simulink library "pack_105s34p_structured"  (R2023b)
settings: Solver=VariableStepAuto  StartTime=0.0  StopTime=10.0  RelTol=1e-3
undefined symbols (not defined in the file or in its folder): battery_builder_rtmsupport, gcbh
libraries: nesl_utility x156, pack_105s34p_structured_lib x156
(part 6 of 7)

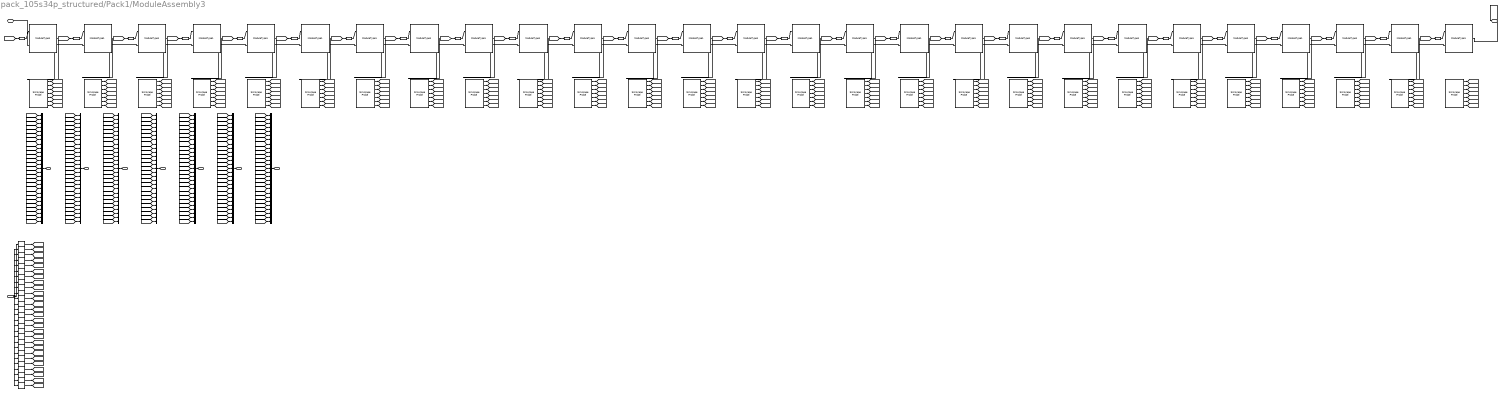
== system pack_105s34p_structured/Pack1/ModuleAssembly3 ==
  note: Balancing Signals
  note: Output Signals
  note: Battery Modules
  balancing : Inport  PortDimensions=27
  Converter{1..27} (27 alike) : nesl_utility/Simulink-PS Converter  PhysicalDomain=network_engine_domain  SubClassName=ps_input  LeftPortType=input  RightPortType=output  PseudoPeriodic=off  Frequencies=[]  NoiseDistribution=none  NoiseParameters=[]  Unit=1  AffineConversion=off  FilteringAndDerivatives=provide  SimscapeFilterOrder=1  InputFilterTimeConstant=0.001  UdotUserProvided=0
  Module01 : pack_105s34p_structured_lib/Modules/ModuleType1  SOC_vecCell=[0, .1, .25, .5, .75, .9, 1]  T_vecCell=[278, 293, 313] K  V0_matCell=[3.49, 3.5, 3.51; 3.55, 3.57, 3.56; 3.62, 3.63, 3.64; 3.71, 3.71, 3.72; 3.91, 3.93, 3.94; 4.07, 4.08, 4.08; 4.19, 4.19, 4.19] V  V_rangeCell=[0, inf] V  R0_matCell=[.0117, .0085, .009; .011, .0085, .009; .0114, .0087, .0092; .0107, .0082, .0088; .0107, .0083, .0091; .0113, .0085, .0089; .0116, .0085, .0089] Ohm  AHCell=4.9 A*hr  extrapolation_optionCell=simscape.enum.extrapolation.nearest  SOC_Init=0  R1_matCell=[.0109, .0029, .0013; .0069, .0024, .0012; .0047, .0026, .0013; .0034, .0016, .001; .0033, .0023, .0014; .0033, .0018, .0011; .0028, .0017, .0011] Ohm  tau1_matCell=[20, 36, 39; 31, 45, 39; 109, 105, 61; 36, 29, 26; 59, 77, 67; 40, 33, 29; 25, 39, 33] s  R2_matCell=[.0109, .0029, .0013; .0069, .0024, .0012; .0047, .0026, .0013; .0034, .0016, .001; .0033, .0023, .0014; .0033, .0018, .0011; .0028, .0017, .0011] Ohm  tau2_matCell=[20, 36, 39; 31, 45, 39; 109, 105, 61; 36, 29, 26; 59, 77, 67; 40, 33, 29; 25, 39, 33] s  R3_matCell=[.0109, .0029, .0013; .0069, .0024, .0012; .0047, .0026, .0013; .0034, .0016, .001; .0033, .0023, .0014; .0033, .0018, .0011; .0028, .0017, .0011] Ohm  tau3_matCell=[20, 36, 39; 31, 45, 39; 109, 105, 61; 36, 29, 26; 59, 77, 67; 40, 33, 29; 25, 39, 33] s  thermal_massCell=100 J/K  CellBalancingClosedResistance=0.01 Ohm  CellBalancingOpenConductance=1e-8 1/Ohm  CellBalancingThreshold=0.5  CellBalancingResistance=50 Ohm  P=34  S=1  iCell_specify=off  iCell_priority=None  iCell=0 A  iCell_nominal_specify=off  iCell_nominal_unit=A  iCell_nominal_value=1  vCell_specify=off  vCell_priority=None  vCell=0 V  vCell_nominal_specify=off  vCell_nominal_unit=V  vCell_nominal_value=1  numCyclesCell_specify=off  numCyclesCell_priority=High  numCyclesCell=0  numCyclesCell_nominal_specify=off  numCyclesCell_nominal_unit=1  numCyclesCell_nominal_value=1  temperatureCell_specify=off  temperatureCell_priority=High  temperatureCell=298.15 K  temperatureCell_nominal_specify=off  temperatureCell_nominal_unit=K  temperatureCell_nominal_value=1  vParallelAssembly_specify=off  vParallelAssembly_priority=None  vParallelAssembly=0 V  vParallelAssembly_nominal_specify=off  vParallelAssembly_nominal_unit=V  vParallelAssembly_nominal_value=1  socParallelAssembly_specify=off  socParallelAssembly_priority=None  socParallelAssembly=1  socParallelAssembly_nominal_specify=off  socParallelAssembly_nominal_unit=1  socParallelAssembly_nominal_value=1
      settings: InternalSimscapePortConfiguration="{\"Bottom\":[{\"id\":\"n\",\"label\":\"-\",\"type\":\"foundation.electrical.electrical\"}],\"Left\":[{\"id\":\"enableCellBalancing\",\"label\":\"CB\",\"type\":\"input\"}],\"Right\":[],\"Top\":[{\"id\":\"p\",\"label\":\"+\",\"type\":\"foundation.electrical.electrical\"}]}"
  Module01_outputs : SimscapeProbe  BoundBlock=2156  Variables={iCell, numCyclesCell, socCell, socParallelAssembly, temperatureCell, vCell, vParallelAssembly}
  Module02 : pack_105s34p_structured_lib/Modules/ModuleType1  SOC_vecCell=[0, .1, .25, .5, .75, .9, 1]  T_vecCell=[278, 293, 313] K  V0_matCell=[3.49, 3.5, 3.51; 3.55, 3.57, 3.56; 3.62, 3.63, 3.64; 3.71, 3.71, 3.72; 3.91, 3.93, 3.94; 4.07, 4.08, 4.08; 4.19, 4.19, 4.19] V  V_rangeCell=[0, inf] V  R0_matCell=[.0117, .0085, .009; .011, .0085, .009; .0114, .0087, .0092; .0107, .0082, .0088; .0107, .0083, .0091; .0113, .0085, .0089; .0116, .0085, .0089] Ohm  AHCell=4.9 A*hr  extrapolation_optionCell=simscape.enum.extrapolation.nearest  SOC_Init=0  R1_matCell=[.0109, .0029, .0013; .0069, .0024, .0012; .0047, .0026, .0013; .0034, .0016, .001; .0033, .0023, .0014; .0033, .0018, .0011; .0028, .0017, .0011] Ohm  tau1_matCell=[20, 36, 39; 31, 45, 39; 109, 105, 61; 36, 29, 26; 59, 77, 67; 40, 33, 29; 25, 39, 33] s  R2_matCell=[.0109, .0029, .0013; .0069, .0024, .0012; .0047, .0026, .0013; .0034, .0016, .001; .0033, .0023, .0014; .0033, .0018, .0011; .0028, .0017, .0011] Ohm  tau2_matCell=[20, 36, 39; 31, 45, 39; 109, 105, 61; 36, 29, 26; 59, 77, 67; 40, 33, 29; 25, 39, 33] s  R3_matCell=[.0109, .0029, .0013; .0069, .0024, .0012; .0047, .0026, .0013; .0034, .0016, .001; .0033, .0023, .0014; .0033, .0018, .0011; .0028, .0017, .0011] Ohm  tau3_matCell=[20, 36, 39; 31, 45, 39; 109, 105, 61; 36, 29, 26; 59, 77, 67; 40, 33, 29; 25, 39, 33] s  thermal_massCell=100 J/K  CellBalancingClosedResistance=0.01 Ohm  CellBalancingOpenConductance=1e-8 1/Ohm  CellBalancingThreshold=0.5  CellBalancingResistance=50 Ohm  P=34  S=1  iCell_specify=off  iCell_priority=None  iCell=0 A  iCell_nominal_specify=off  iCell_nominal_unit=A  iCell_nominal_value=1  vCell_specify=off  vCell_priority=None  vCell=0 V  vCell_nominal_specify=off  vCell_nominal_unit=V  vCell_nominal_value=1  numCyclesCell_specify=off  numCyclesCell_priority=High  numCyclesCell=0  numCyclesCell_nominal_specify=off  numCyclesCell_nominal_unit=1  numCyclesCell_nominal_value=1  temperatureCell_specify=off  temperatureCell_priority=High  temperatureCell=298.15 K  temperatureCell_nominal_specify=off  temperatureCell_nominal_unit=K  temperatureCell_nominal_value=1  vParallelAssembly_specify=off  vParallelAssembly_priority=None  vParallelAssembly=0 V  vParallelAssembly_nominal_specify=off  vParallelAssembly_nominal_unit=V  vParallelAssembly_nominal_value=1  socParallelAssembly_specify=off  socParallelAssembly_priority=None  socParallelAssembly=1  socParallelAssembly_nominal_specify=off  socParallelAssembly_nominal_unit=1  socParallelAssembly_nominal_value=1
      settings: InternalSimscapePortConfiguration="{\"Bottom\":[{\"id\":\"n\",\"label\":\"-\",\"type\":\"foundation.electrical.electrical\"}],\"Left\":[{\"id\":\"enableCellBalancing\",\"label\":\"CB\",\"type\":\"input\"}],\"Right\":[],\"Top\":[{\"id\":\"p\",\"label\":\"+\",\"type\":\"foundation.electrical.electrical\"}]}"
  Module02_outputs : SimscapeProbe  BoundBlock=2158  Variables={iCell, numCyclesCell, socCell, socParallelAssembly, temperatureCell, vCell, vParallelAssembly}
  Module03 : pack_105s34p_structured_lib/Modules/ModuleType1  SOC_vecCell=[0, .1, .25, .5, .75, .9, 1]  T_vecCell=[278, 293, 313] K  V0_matCell=[3.49, 3.5, 3.51; 3.55, 3.57, 3.56; 3.62, 3.63, 3.64; 3.71, 3.71, 3.72; 3.91, 3.93, 3.94; 4.07, 4.08, 4.08; 4.19, 4.19, 4.19] V  V_rangeCell=[0, inf] V  R0_matCell=[.0117, .0085, .009; .011, .0085, .009; .0114, .0087, .0092; .0107, .0082, .0088; .0107, .0083, .0091; .0113, .0085, .0089; .0116, .0085, .0089] Ohm  AHCell=4.9 A*hr  extrapolation_optionCell=simscape.enum.extrapolation.nearest  SOC_Init=0  R1_matCell=[.0109, .0029, .0013; .0069, .0024, .0012; .0047, .0026, .0013; .0034, .0016, .001; .0033, .0023, .0014; .0033, .0018, .0011; .0028, .0017, .0011] Ohm  tau1_matCell=[20, 36, 39; 31, 45, 39; 109, 105, 61; 36, 29, 26; 59, 77, 67; 40, 33, 29; 25, 39, 33] s  R2_matCell=[.0109, .0029, .0013; .0069, .0024, .0012; .0047, .0026, .0013; .0034, .0016, .001; .0033, .0023, .0014; .0033, .0018, .0011; .0028, .0017, .0011] Ohm  tau2_matCell=[20, 36, 39; 31, 45, 39; 109, 105, 61; 36, 29, 26; 59, 77, 67; 40, 33, 29; 25, 39, 33] s  R3_matCell=[.0109, .0029, .0013; .0069, .0024, .0012; .0047, .0026, .0013; .0034, .0016, .001; .0033, .0023, .0014; .0033, .0018, .0011; .0028, .0017, .0011] Ohm  tau3_matCell=[20, 36, 39; 31, 45, 39; 109, 105, 61; 36, 29, 26; 59, 77, 67; 40, 33, 29; 25, 39, 33] s  thermal_massCell=100 J/K  CellBalancingClosedResistance=0.01 Ohm  CellBalancingOpenConductance=1e-8 1/Ohm  CellBalancingThreshold=0.5  CellBalancingResistance=50 Ohm  P=34  S=1  iCell_specify=off  iCell_priority=None  iCell=0 A  iCell_nominal_specify=off  iCell_nominal_unit=A  iCell_nominal_value=1  vCell_specify=off  vCell_priority=None  vCell=0 V  vCell_nominal_specify=off  vCell_nominal_unit=V  vCell_nominal_value=1  numCyclesCell_specify=off  numCyclesCell_priority=High  numCyclesCell=0  numCyclesCell_nominal_specify=off  numCyclesCell_nominal_unit=1  numCyclesCell_nominal_value=1  temperatureCell_specify=off  temperatureCell_priority=High  temperatureCell=298.15 K  temperatureCell_nominal_specify=off  temperatureCell_nominal_unit=K  temperatureCell_nominal_value=1  vParallelAssembly_specify=off  vParallelAssembly_priority=None  vParallelAssembly=0 V  vParallelAssembly_nominal_specify=off  vParallelAssembly_nominal_unit=V  vParallelAssembly_nominal_value=1  socParallelAssembly_specify=off  socParallelAssembly_priority=None  socParallelAssembly=1  socParallelAssembly_nominal_specify=off  socParallelAssembly_nominal_unit=1  socParallelAssembly_nominal_value=1
      settings: InternalSimscapePortConfiguration="{\"Bottom\":[{\"id\":\"n\",\"label\":\"-\",\"type\":\"foundation.electrical.electrical\"}],\"Left\":[{\"id\":\"enableCellBalancing\",\"label\":\"CB\",\"type\":\"input\"}],\"Right\":[],\"Top\":[{\"id\":\"p\",\"label\":\"+\",\"type\":\"foundation.electrical.electrical\"}]}"
  Module03_outputs : SimscapeProbe  BoundBlock=2160  Variables={iCell, numCyclesCell, socCell, socParallelAssembly, temperatureCell, vCell, vParallelAssembly}
  Module04 : pack_105s34p_structured_lib/Modules/ModuleType1  SOC_vecCell=[0, .1, .25, .5, .75, .9, 1]  T_vecCell=[278, 293, 313] K  V0_matCell=[3.49, 3.5, 3.51; 3.55, 3.57, 3.56; 3.62, 3.63, 3.64; 3.71, 3.71, 3.72; 3.91, 3.93, 3.94; 4.07, 4.08, 4.08; 4.19, 4.19, 4.19] V  V_rangeCell=[0, inf] V  R0_matCell=[.0117, .0085, .009; .011, .0085, .009; .0114, .0087, .0092; .0107, .0082, .0088; .0107, .0083, .0091; .0113, .0085, .0089; .0116, .0085, .0089] Ohm  AHCell=4.9 A*hr  extrapolation_optionCell=simscape.enum.extrapolation.nearest  SOC_Init=0  R1_matCell=[.0109, .0029, .0013; .0069, .0024, .0012; .0047, .0026, .0013; .0034, .0016, .001; .0033, .0023, .0014; .0033, .0018, .0011; .0028, .0017, .0011] Ohm  tau1_matCell=[20, 36, 39; 31, 45, 39; 109, 105, 61; 36, 29, 26; 59, 77, 67; 40, 33, 29; 25, 39, 33] s  R2_matCell=[.0109, .0029, .0013; .0069, .0024, .0012; .0047, .0026, .0013; .0034, .0016, .001; .0033, .0023, .0014; .0033, .0018, .0011; .0028, .0017, .0011] Ohm  tau2_matCell=[20, 36, 39; 31, 45, 39; 109, 105, 61; 36, 29, 26; 59, 77, 67; 40, 33, 29; 25, 39, 33] s  R3_matCell=[.0109, .0029, .0013; .0069, .0024, .0012; .0047, .0026, .0013; .0034, .0016, .001; .0033, .0023, .0014; .0033, .0018, .0011; .0028, .0017, .0011] Ohm  tau3_matCell=[20, 36, 39; 31, 45, 39; 109, 105, 61; 36, 29, 26; 59, 77, 67; 40, 33, 29; 25, 39, 33] s  thermal_massCell=100 J/K  CellBalancingClosedResistance=0.01 Ohm  CellBalancingOpenConductance=1e-8 1/Ohm  CellBalancingThreshold=0.5  CellBalancingResistance=50 Ohm  P=34  S=1  iCell_specify=off  iCell_priority=None  iCell=0 A  iCell_nominal_specify=off  iCell_nominal_unit=A  iCell_nominal_value=1  vCell_specify=off  vCell_priority=None  vCell=0 V  vCell_nominal_specify=off  vCell_nominal_unit=V  vCell_nominal_value=1  numCyclesCell_specify=off  numCyclesCell_priority=High  numCyclesCell=0  numCyclesCell_nominal_specify=off  numCyclesCell_nominal_unit=1  numCyclesCell_nominal_value=1  temperatureCell_specify=off  temperatureCell_priority=High  temperatureCell=298.15 K  temperatureCell_nominal_specify=off  temperatureCell_nominal_unit=K  temperatureCell_nominal_value=1  vParallelAssembly_specify=off  vParallelAssembly_priority=None  vParallelAssembly=0 V  vParallelAssembly_nominal_specify=off  vParallelAssembly_nominal_unit=V  vParallelAssembly_nominal_value=1  socParallelAssembly_specify=off  socParallelAssembly_priority=None  socParallelAssembly=1  socParallelAssembly_nominal_specify=off  socParallelAssembly_nominal_unit=1  socParallelAssembly_nominal_value=1
      settings: InternalSimscapePortConfiguration="{\"Bottom\":[{\"id\":\"n\",\"label\":\"-\",\"type\":\"foundation.electrical.electrical\"}],\"Left\":[{\"id\":\"enableCellBalancing\",\"label\":\"CB\",\"type\":\"input\"}],\"Right\":[],\"Top\":[{\"id\":\"p\",\"label\":\"+\",\"type\":\"foundation.electrical.electrical\"}]}"
  Module04_outputs : SimscapeProbe  BoundBlock=2162  Variables={iCell, numCyclesCell, socCell, socParallelAssembly, temperatureCell, vCell, vParallelAssembly}
  Module05 : pack_105s34p_structured_lib/Modules/ModuleType1  SOC_vecCell=[0, .1, .25, .5, .75, .9, 1]  T_vecCell=[278, 293, 313] K  V0_matCell=[3.49, 3.5, 3.51; 3.55, 3.57, 3.56; 3.62, 3.63, 3.64; 3.71, 3.71, 3.72; 3.91, 3.93, 3.94; 4.07, 4.08, 4.08; 4.19, 4.19, 4.19] V  V_rangeCell=[0, inf] V  R0_matCell=[.0117, .0085, .009; .011, .0085, .009; .0114, .0087, .0092; .0107, .0082, .0088; .0107, .0083, .0091; .0113, .0085, .0089; .0116, .0085, .0089] Ohm  AHCell=4.9 A*hr  extrapolation_optionCell=simscape.enum.extrapolation.nearest  SOC_Init=0  R1_matCell=[.0109, .0029, .0013; .0069, .0024, .0012; .0047, .0026, .0013; .0034, .0016, .001; .0033, .0023, .0014; .0033, .0018, .0011; .0028, .0017, .0011] Ohm  tau1_matCell=[20, 36, 39; 31, 45, 39; 109, 105, 61; 36, 29, 26; 59, 77, 67; 40, 33, 29; 25, 39, 33] s  R2_matCell=[.0109, .0029, .0013; .0069, .0024, .0012; .0047, .0026, .0013; .0034, .0016, .001; .0033, .0023, .0014; .0033, .0018, .0011; .0028, .0017, .0011] Ohm  tau2_matCell=[20, 36, 39; 31, 45, 39; 109, 105, 61; 36, 29, 26; 59, 77, 67; 40, 33, 29; 25, 39, 33] s  R3_matCell=[.0109, .0029, .0013; .0069, .0024, .0012; .0047, .0026, .0013; .0034, .0016, .001; .0033, .0023, .0014; .0033, .0018, .0011; .0028, .0017, .0011] Ohm  tau3_matCell=[20, 36, 39; 31, 45, 39; 109, 105, 61; 36, 29, 26; 59, 77, 67; 40, 33, 29; 25, 39, 33] s  thermal_massCell=100 J/K  CellBalancingClosedResistance=0.01 Ohm  CellBalancingOpenConductance=1e-8 1/Ohm  CellBalancingThreshold=0.5  CellBalancingResistance=50 Ohm  P=34  S=1  iCell_specify=off  iCell_priority=None  iCell=0 A  iCell_nominal_specify=off  iCell_nominal_unit=A  iCell_nominal_value=1  vCell_specify=off  vCell_priority=None  vCell=0 V  vCell_nominal_specify=off  vCell_nominal_unit=V  vCell_nominal_value=1  numCyclesCell_specify=off  numCyclesCell_priority=High  numCyclesCell=0  numCyclesCell_nominal_specify=off  numCyclesCell_nominal_unit=1  numCyclesCell_nominal_value=1  temperatureCell_specify=off  temperatureCell_priority=High  temperatureCell=298.15 K  temperatureCell_nominal_specify=off  temperatureCell_nominal_unit=K  temperatureCell_nominal_value=1  vParallelAssembly_specify=off  vParallelAssembly_priority=None  vParallelAssembly=0 V  vParallelAssembly_nominal_specify=off  vParallelAssembly_nominal_unit=V  vParallelAssembly_nominal_value=1  socParallelAssembly_specify=off  socParallelAssembly_priority=None  socParallelAssembly=1  socParallelAssembly_nominal_specify=off  socParallelAssembly_nominal_unit=1  socParallelAssembly_nominal_value=1
      settings: InternalSimscapePortConfiguration="{\"Bottom\":[{\"id\":\"n\",\"label\":\"-\",\"type\":\"foundation.electrical.electrical\"}],\"Left\":[{\"id\":\"enableCellBalancing\",\"label\":\"CB\",\"type\":\"input\"}],\"Right\":[],\"Top\":[{\"id\":\"p\",\"label\":\"+\",\"type\":\"foundation.electrical.electrical\"}]}"
  Module05_outputs : SimscapeProbe  BoundBlock=2164  Variables={iCell, numCyclesCell, socCell, socParallelAssembly, temperatureCell, vCell, vParallelAssembly}
  Module06 : pack_105s34p_structured_lib/Modules/ModuleType1  SOC_vecCell=[0, .1, .25, .5, .75, .9, 1]  T_vecCell=[278, 293, 313] K  V0_matCell=[3.49, 3.5, 3.51; 3.55, 3.57, 3.56; 3.62, 3.63, 3.64; 3.71, 3.71, 3.72; 3.91, 3.93, 3.94; 4.07, 4.08, 4.08; 4.19, 4.19, 4.19] V  V_rangeCell=[0, inf] V  R0_matCell=[.0117, .0085, .009; .011, .0085, .009; .0114, .0087, .0092; .0107, .0082, .0088; .0107, .0083, .0091; .0113, .0085, .0089; .0116, .0085, .0089] Ohm  AHCell=4.9 A*hr  extrapolation_optionCell=simscape.enum.extrapolation.nearest  SOC_Init=0  R1_matCell=[.0109, .0029, .0013; .0069, .0024, .0012; .0047, .0026, .0013; .0034, .0016, .001; .0033, .0023, .0014; .0033, .0018, .0011; .0028, .0017, .0011] Ohm  tau1_matCell=[20, 36, 39; 31, 45, 39; 109, 105, 61; 36, 29, 26; 59, 77, 67; 40, 33, 29; 25, 39, 33] s  R2_matCell=[.0109, .0029, .0013; .0069, .0024, .0012; .0047, .0026, .0013; .0034, .0016, .001; .0033, .0023, .0014; .0033, .0018, .0011; .0028, .0017, .0011] Ohm  tau2_matCell=[20, 36, 39; 31, 45, 39; 109, 105, 61; 36, 29, 26; 59, 77, 67; 40, 33, 29; 25, 39, 33] s  R3_matCell=[.0109, .0029, .0013; .0069, .0024, .0012; .0047, .0026, .0013; .0034, .0016, .001; .0033, .0023, .0014; .0033, .0018, .0011; .0028, .0017, .0011] Ohm  tau3_matCell=[20, 36, 39; 31, 45, 39; 109, 105, 61; 36, 29, 26; 59, 77, 67; 40, 33, 29; 25, 39, 33] s  thermal_massCell=100 J/K  CellBalancingClosedResistance=0.01 Ohm  CellBalancingOpenConductance=1e-8 1/Ohm  CellBalancingThreshold=0.5  CellBalancingResistance=50 Ohm  P=34  S=1  iCell_specify=off  iCell_priority=None  iCell=0 A  iCell_nominal_specify=off  iCell_nominal_unit=A  iCell_nominal_value=1  vCell_specify=off  vCell_priority=None  vCell=0 V  vCell_nominal_specify=off  vCell_nominal_unit=V  vCell_nominal_value=1  numCyclesCell_specify=off  numCyclesCell_priority=High  numCyclesCell=0  numCyclesCell_nominal_specify=off  numCyclesCell_nominal_unit=1  numCyclesCell_nominal_value=1  temperatureCell_specify=off  temperatureCell_priority=High  temperatureCell=298.15 K  temperatureCell_nominal_specify=off  temperatureCell_nominal_unit=K  temperatureCell_nominal_value=1  vParallelAssembly_specify=off  vParallelAssembly_priority=None  vParallelAssembly=0 V  vParallelAssembly_nominal_specify=off  vParallelAssembly_nominal_unit=V  vParallelAssembly_nominal_value=1  socParallelAssembly_specify=off  socParallelAssembly_priority=None  socParallelAssembly=1  socParallelAssembly_nominal_specify=off  socParallelAssembly_nominal_unit=1  socParallelAssembly_nominal_value=1
      settings: InternalSimscapePortConfiguration="{\"Bottom\":[{\"id\":\"n\",\"label\":\"-\",\"type\":\"foundation.electrical.electrical\"}],\"Left\":[{\"id\":\"enableCellBalancing\",\"label\":\"CB\",\"type\":\"input\"}],\"Right\":[],\"Top\":[{\"id\":\"p\",\"label\":\"+\",\"type\":\"foundation.electrical.electrical\"}]}"
  Module06_outputs : SimscapeProbe  BoundBlock=2166  Variables={iCell, numCyclesCell, socCell, socParallelAssembly, temperatureCell, vCell, vParallelAssembly}
  Module07 : pack_105s34p_structured_lib/Modules/ModuleType1  SOC_vecCell=[0, .1, .25, .5, .75, .9, 1]  T_vecCell=[278, 293, 313] K  V0_matCell=[3.49, 3.5, 3.51; 3.55, 3.57, 3.56; 3.62, 3.63, 3.64; 3.71, 3.71, 3.72; 3.91, 3.93, 3.94; 4.07, 4.08, 4.08; 4.19, 4.19, 4.19] V  V_rangeCell=[0, inf] V  R0_matCell=[.0117, .0085, .009; .011, .0085, .009; .0114, .0087, .0092; .0107, .0082, .0088; .0107, .0083, .0091; .0113, .0085, .0089; .0116, .0085, .0089] Ohm  AHCell=4.9 A*hr  extrapolation_optionCell=simscape.enum.extrapolation.nearest  SOC_Init=0  R1_matCell=[.0109, .0029, .0013; .0069, .0024, .0012; .0047, .0026, .0013; .0034, .0016, .001; .0033, .0023, .0014; .0033, .0018, .0011; .0028, .0017, .0011] Ohm  tau1_matCell=[20, 36, 39; 31, 45, 39; 109, 105, 61; 36, 29, 26; 59, 77, 67; 40, 33, 29; 25, 39, 33] s  R2_matCell=[.0109, .0029, .0013; .0069, .0024, .0012; .0047, .0026, .0013; .0034, .0016, .001; .0033, .0023, .0014; .0033, .0018, .0011; .0028, .0017, .0011] Ohm  tau2_matCell=[20, 36, 39; 31, 45, 39; 109, 105, 61; 36, 29, 26; 59, 77, 67; 40, 33, 29; 25, 39, 33] s  R3_matCell=[.0109, .0029, .0013; .0069, .0024, .0012; .0047, .0026, .0013; .0034, .0016, .001; .0033, .0023, .0014; .0033, .0018, .0011; .0028, .0017, .0011] Ohm  tau3_matCell=[20, 36, 39; 31, 45, 39; 109, 105, 61; 36, 29, 26; 59, 77, 67; 40, 33, 29; 25, 39, 33] s  thermal_massCell=100 J/K  CellBalancingClosedResistance=0.01 Ohm  CellBalancingOpenConductance=1e-8 1/Ohm  CellBalancingThreshold=0.5  CellBalancingResistance=50 Ohm  P=34  S=1  iCell_specify=off  iCell_priority=None  iCell=0 A  iCell_nominal_specify=off  iCell_nominal_unit=A  iCell_nominal_value=1  vCell_specify=off  vCell_priority=None  vCell=0 V  vCell_nominal_specify=off  vCell_nominal_unit=V  vCell_nominal_value=1  numCyclesCell_specify=off  numCyclesCell_priority=High  numCyclesCell=0  numCyclesCell_nominal_specify=off  numCyclesCell_nominal_unit=1  numCyclesCell_nominal_value=1  temperatureCell_specify=off  temperatureCell_priority=High  temperatureCell=298.15 K  temperatureCell_nominal_specify=off  temperatureCell_nominal_unit=K  temperatureCell_nominal_value=1  vParallelAssembly_specify=off  vParallelAssembly_priority=None  vParallelAssembly=0 V  vParallelAssembly_nominal_specify=off  vParallelAssembly_nominal_unit=V  vParallelAssembly_nominal_value=1  socParallelAssembly_specify=off  socParallelAssembly_priority=None  socParallelAssembly=1  socParallelAssembly_nominal_specify=off  socParallelAssembly_nominal_unit=1  socParallelAssembly_nominal_value=1
      settings: InternalSimscapePortConfiguration="{\"Bottom\":[{\"id\":\"n\",\"label\":\"-\",\"type\":\"foundation.electrical.electrical\"}],\"Left\":[{\"id\":\"enableCellBalancing\",\"label\":\"CB\",\"type\":\"input\"}],\"Right\":[],\"Top\":[{\"id\":\"p\",\"label\":\"+\",\"type\":\"foundation.electrical.electrical\"}]}"
  Module07_outputs : SimscapeProbe  BoundBlock=2168  Variables={iCell, numCyclesCell, socCell, socParallelAssembly, temperatureCell, vCell, vParallelAssembly}
  Module08 : pack_105s34p_structured_lib/Modules/ModuleType1  SOC_vecCell=[0, .1, .25, .5, .75, .9, 1]  T_vecCell=[278, 293, 313] K  V0_matCell=[3.49, 3.5, 3.51; 3.55, 3.57, 3.56; 3.62, 3.63, 3.64; 3.71, 3.71, 3.72; 3.91, 3.93, 3.94; 4.07, 4.08, 4.08; 4.19, 4.19, 4.19] V  V_rangeCell=[0, inf] V  R0_matCell=[.0117, .0085, .009; .011, .0085, .009; .0114, .0087, .0092; .0107, .0082, .0088; .0107, .0083, .0091; .0113, .0085, .0089; .0116, .0085, .0089] Ohm  AHCell=4.9 A*hr  extrapolation_optionCell=simscape.enum.extrapolation.nearest  SOC_Init=0  R1_matCell=[.0109, .0029, .0013; .0069, .0024, .0012; .0047, .0026, .0013; .0034, .0016, .001; .0033, .0023, .0014; .0033, .0018, .0011; .0028, .0017, .0011] Ohm  tau1_matCell=[20, 36, 39; 31, 45, 39; 109, 105, 61; 36, 29, 26; 59, 77, 67; 40, 33, 29; 25, 39, 33] s  R2_matCell=[.0109, .0029, .0013; .0069, .0024, .0012; .0047, .0026, .0013; .0034, .0016, .001; .0033, .0023, .0014; .0033, .0018, .0011; .0028, .0017, .0011] Ohm  tau2_matCell=[20, 36, 39; 31, 45, 39; 109, 105, 61; 36, 29, 26; 59, 77, 67; 40, 33, 29; 25, 39, 33] s  R3_matCell=[.0109, .0029, .0013; .0069, .0024, .0012; .0047, .0026, .0013; .0034, .0016, .001; .0033, .0023, .0014; .0033, .0018, .0011; .0028, .0017, .0011] Ohm  tau3_matCell=[20, 36, 39; 31, 45, 39; 109, 105, 61; 36, 29, 26; 59, 77, 67; 40, 33, 29; 25, 39, 33] s  thermal_massCell=100 J/K  CellBalancingClosedResistance=0.01 Ohm  CellBalancingOpenConductance=1e-8 1/Ohm  CellBalancingThreshold=0.5  CellBalancingResistance=50 Ohm  P=34  S=1  iCell_specify=off  iCell_priority=None  iCell=0 A  iCell_nominal_specify=off  iCell_nominal_unit=A  iCell_nominal_value=1  vCell_specify=off  vCell_priority=None  vCell=0 V  vCell_nominal_specify=off  vCell_nominal_unit=V  vCell_nominal_value=1  numCyclesCell_specify=off  numCyclesCell_priority=High  numCyclesCell=0  numCyclesCell_nominal_specify=off  numCyclesCell_nominal_unit=1  numCyclesCell_nominal_value=1  temperatureCell_specify=off  temperatureCell_priority=High  temperatureCell=298.15 K  temperatureCell_nominal_specify=off  temperatureCell_nominal_unit=K  temperatureCell_nominal_value=1  vParallelAssembly_specify=off  vParallelAssembly_priority=None  vParallelAssembly=0 V  vParallelAssembly_nominal_specify=off  vParallelAssembly_nominal_unit=V  vParallelAssembly_nominal_value=1  socParallelAssembly_specify=off  socParallelAssembly_priority=None  socParallelAssembly=1  socParallelAssembly_nominal_specify=off  socParallelAssembly_nominal_unit=1  socParallelAssembly_nominal_value=1
      settings: InternalSimscapePortConfiguration="{\"Bottom\":[{\"id\":\"n\",\"label\":\"-\",\"type\":\"foundation.electrical.electrical\"}],\"Left\":[{\"id\":\"enableCellBalancing\",\"label\":\"CB\",\"type\":\"input\"}],\"Right\":[],\"Top\":[{\"id\":\"p\",\"label\":\"+\",\"type\":\"foundation.electrical.electrical\"}]}"
  Module08_outputs : SimscapeProbe  BoundBlock=2170  Variables={iCell, numCyclesCell, socCell, socParallelAssembly, temperatureCell, vCell, vParallelAssembly}
  Module09 : pack_105s34p_structured_lib/Modules/ModuleType1  SOC_vecCell=[0, .1, .25, .5, .75, .9, 1]  T_vecCell=[278, 293, 313] K  V0_matCell=[3.49, 3.5, 3.51; 3.55, 3.57, 3.56; 3.62, 3.63, 3.64; 3.71, 3.71, 3.72; 3.91, 3.93, 3.94; 4.07, 4.08, 4.08; 4.19, 4.19, 4.19] V  V_rangeCell=[0, inf] V  R0_matCell=[.0117, .0085, .009; .011, .0085, .009; .0114, .0087, .0092; .0107, .0082, .0088; .0107, .0083, .0091; .0113, .0085, .0089; .0116, .0085, .0089] Ohm  AHCell=4.9 A*hr  extrapolation_optionCell=simscape.enum.extrapolation.nearest  SOC_Init=0  R1_matCell=[.0109, .0029, .0013; .0069, .0024, .0012; .0047, .0026, .0013; .0034, .0016, .001; .0033, .0023, .0014; .0033, .0018, .0011; .0028, .0017, .0011] Ohm  tau1_matCell=[20, 36, 39; 31, 45, 39; 109, 105, 61; 36, 29, 26; 59, 77, 67; 40, 33, 29; 25, 39, 33] s  R2_matCell=[.0109, .0029, .0013; .0069, .0024, .0012; .0047, .0026, .0013; .0034, .0016, .001; .0033, .0023, .0014; .0033, .0018, .0011; .0028, .0017, .0011] Ohm  tau2_matCell=[20, 36, 39; 31, 45, 39; 109, 105, 61; 36, 29, 26; 59, 77, 67; 40, 33, 29; 25, 39, 33] s  R3_matCell=[.0109, .0029, .0013; .0069, .0024, .0012; .0047, .0026, .0013; .0034, .0016, .001; .0033, .0023, .0014; .0033, .0018, .0011; .0028, .0017, .0011] Ohm  tau3_matCell=[20, 36, 39; 31, 45, 39; 109, 105, 61; 36, 29, 26; 59, 77, 67; 40, 33, 29; 25, 39, 33] s  thermal_massCell=100 J/K  CellBalancingClosedResistance=0.01 Ohm  CellBalancingOpenConductance=1e-8 1/Ohm  CellBalancingThreshold=0.5  CellBalancingResistance=50 Ohm  P=34  S=1  iCell_specify=off  iCell_priority=None  iCell=0 A  iCell_nominal_specify=off  iCell_nominal_unit=A  iCell_nominal_value=1  vCell_specify=off  vCell_priority=None  vCell=0 V  vCell_nominal_specify=off  vCell_nominal_unit=V  vCell_nominal_value=1  numCyclesCell_specify=off  numCyclesCell_priority=High  numCyclesCell=0  numCyclesCell_nominal_specify=off  numCyclesCell_nominal_unit=1  numCyclesCell_nominal_value=1  temperatureCell_specify=off  temperatureCell_priority=High  temperatureCell=298.15 K  temperatureCell_nominal_specify=off  temperatureCell_nominal_unit=K  temperatureCell_nominal_value=1  vParallelAssembly_specify=off  vParallelAssembly_priority=None  vParallelAssembly=0 V  vParallelAssembly_nominal_specify=off  vParallelAssembly_nominal_unit=V  vParallelAssembly_nominal_value=1  socParallelAssembly_specify=off  socParallelAssembly_priority=None  socParallelAssembly=1  socParallelAssembly_nominal_specify=off  socParallelAssembly_nominal_unit=1  socParallelAssembly_nominal_value=1
      settings: InternalSimscapePortConfiguration="{\"Bottom\":[{\"id\":\"n\",\"label\":\"-\",\"type\":\"foundation.electrical.electrical\"}],\"Left\":[{\"id\":\"enableCellBalancing\",\"label\":\"CB\",\"type\":\"input\"}],\"Right\":[],\"Top\":[{\"id\":\"p\",\"label\":\"+\",\"type\":\"foundation.electrical.electrical\"}]}"
  Module09_outputs : SimscapeProbe  BoundBlock=2172  Variables={iCell, numCyclesCell, socCell, socParallelAssembly, temperatureCell, vCell, vParallelAssembly}
  Module{10..27} (18 alike) : pack_105s34p_structured_lib/Modules/ModuleType1  SOC_vecCell=[0, .1, .25, .5, .75, .9, 1]  T_vecCell=[278, 293, 313] K  V0_matCell=[3.49, 3.5, 3.51; 3.55, 3.57, 3.56; 3.62, 3.63, 3.64; 3.71, 3.71, 3.72; 3.91, 3.93, 3.94; 4.07, 4.08, 4.08; 4.19, 4.19, 4.19] V  V_rangeCell=[0, inf] V  R0_matCell=[.0117, .0085, .009; .011, .0085, .009; .0114, .0087, .0092; .0107, .0082, .0088; .0107, .0083, .0091; .0113, .0085, .0089; .0116, .0085, .0089] Ohm  AHCell=4.9 A*hr  extrapolation_optionCell=simscape.enum.extrapolation.nearest  SOC_Init=0  R1_matCell=[.0109, .0029, .0013; .0069, .0024, .0012; .0047, .0026, .0013; .0034, .0016, .001; .0033, .0023, .0014; .0033, .0018, .0011; .0028, .0017, .0011] Ohm  tau1_matCell=[20, 36, 39; 31, 45, 39; 109, 105, 61; 36, 29, 26; 59, 77, 67; 40, 33, 29; 25, 39, 33] s  R2_matCell=[.0109, .0029, .0013; .0069, .0024, .0012; .0047, .0026, .0013; .0034, .0016, .001; .0033, .0023, .0014; .0033, .0018, .0011; .0028, .0017, .0011] Ohm  tau2_matCell=[20, 36, 39; 31, 45, 39; 109, 105, 61; 36, 29, 26; 59, 77, 67; 40, 33, 29; 25, 39, 33] s  R3_matCell=[.0109, .0029, .0013; .0069, .0024, .0012; .0047, .0026, .0013; .0034, .0016, .001; .0033, .0023, .0014; .0033, .0018, .0011; .0028, .0017, .0011] Ohm  tau3_matCell=[20, 36, 39; 31, 45, 39; 109, 105, 61; 36, 29, 26; 59, 77, 67; 40, 33, 29; 25, 39, 33] s  thermal_massCell=100 J/K  CellBalancingClosedResistance=0.01 Ohm  CellBalancingOpenConductance=1e-8 1/Ohm  CellBalancingThreshold=0.5  CellBalancingResistance=50 Ohm  P=34  S=1  iCell_specify=off  iCell_priority=None  iCell=0 A  iCell_nominal_specify=off  iCell_nominal_unit=A  iCell_nominal_value=1  vCell_specify=off  vCell_priority=None  vCell=0 V  vCell_nominal_specify=off  vCell_nominal_unit=V  vCell_nominal_value=1  numCyclesCell_specify=off  numCyclesCell_priority=High  numCyclesCell=0  numCyclesCell_nominal_specify=off  numCyclesCell_nominal_unit=1  numCyclesCell_nominal_value=1  temperatureCell_specify=off  temperatureCell_priority=High  temperatureCell=298.15 K  temperatureCell_nominal_specify=off  temperatureCell_nominal_unit=K  temperatureCell_nominal_value=1  vParallelAssembly_specify=off  vParallelAssembly_priority=None  vParallelAssembly=0 V  vParallelAssembly_nominal_specify=off  vParallelAssembly_nominal_unit=V  vParallelAssembly_nominal_value=1  socParallelAssembly_specify=off  socParallelAssembly_priority=None  socParallelAssembly=1  socParallelAssembly_nominal_specify=off  socParallelAssembly_nominal_unit=1  socParallelAssembly_nominal_value=1
      settings: InternalSimscapePortConfiguration="{\"Bottom\":[{\"id\":\"n\",\"label\":\"-\",\"type\":\"foundation.electrical.electrical\"}],\"Left\":[{\"id\":\"enableCellBalancing\",\"label\":\"CB\",\"type\":\"input\"}],\"Right\":[],\"Top\":[{\"id\":\"p\",\"label\":\"+\",\"type\":\"foundation.electrical.electrical\"}]}"
  Module10_outputs : SimscapeProbe  BoundBlock=2174  Variables={iCell, numCyclesCell, socCell, socParallelAssembly, temperatureCell, vCell, vParallelAssembly}
  Module11_outputs : SimscapeProbe  BoundBlock=2176  Variables={iCell, numCyclesCell, socCell, socParallelAssembly, temperatureCell, vCell, vParallelAssembly}
  Module12_outputs : SimscapeProbe  BoundBlock=2178  Variables={iCell, numCyclesCell, socCell, socParallelAssembly, temperatureCell, vCell, vParallelAssembly}
  Module13_outputs : SimscapeProbe  BoundBlock=2180  Variables={iCell, numCyclesCell, socCell, socParallelAssembly, temperatureCell, vCell, vParallelAssembly}
  Module14_outputs : SimscapeProbe  BoundBlock=2182  Variables={iCell, numCyclesCell, socCell, socParallelAssembly, temperatureCell, vCell, vParallelAssembly}
  Module15_outputs : SimscapeProbe  BoundBlock=2184  Variables={iCell, numCyclesCell, socCell, socParallelAssembly, temperatureCell, vCell, vParallelAssembly}
  Module16_outputs : SimscapeProbe  BoundBlock=2186  Variables={iCell, numCyclesCell, socCell, socParallelAssembly, temperatureCell, vCell, vParallelAssembly}
  Module17_outputs : SimscapeProbe  BoundBlock=2188  Variables={iCell, numCyclesCell, socCell, socParallelAssembly, temperatureCell, vCell, vParallelAssembly}
  Module18_outputs : SimscapeProbe  BoundBlock=2190  Variables={iCell, numCyclesCell, socCell, socParallelAssembly, temperatureCell, vCell, vParallelAssembly}
  Module19_outputs : SimscapeProbe  BoundBlock=2192  Variables={iCell, numCyclesCell, socCell, socParallelAssembly, temperatureCell, vCell, vParallelAssembly}
  Module20_outputs : SimscapeProbe  BoundBlock=2194  Variables={iCell, numCyclesCell, socCell, socParallelAssembly, temperatureCell, vCell, vParallelAssembly}
  Module21_outputs : SimscapeProbe  BoundBlock=2196  Variables={iCell, numCyclesCell, socCell, socParallelAssembly, temperatureCell, vCell, vParallelAssembly}
  Module22_outputs : SimscapeProbe  BoundBlock=2198  Variables={iCell, numCyclesCell, socCell, socParallelAssembly, temperatureCell, vCell, vParallelAssembly}
  Module23_outputs : SimscapeProbe  BoundBlock=2200  Variables={iCell, numCyclesCell, socCell, socParallelAssembly, temperatureCell, vCell, vParallelAssembly}
  Module24_outputs : SimscapeProbe  BoundBlock=2202  Variables={iCell, numCyclesCell, socCell, socParallelAssembly, temperatureCell, vCell, vParallelAssembly}
  Module25_outputs : SimscapeProbe  BoundBlock=2204  Variables={iCell, numCyclesCell, socCell, socParallelAssembly, temperatureCell, vCell, vParallelAssembly}
  Module26_outputs : SimscapeProbe  BoundBlock=2206  Variables={iCell, numCyclesCell, socCell, socParallelAssembly, temperatureCell, vCell, vParallelAssembly}
  Module27_outputs : SimscapeProbe  BoundBlock=2208  Variables={iCell, numCyclesCell, socCell, socParallelAssembly, temperatureCell, vCell, vParallelAssembly}
  balancingSelector1 : Selector  InputPortWidth=27  IndexOptions=Index vector (dialog)  Indices=[1]  OutputSizes=1
  balancingSelector10 : Selector  InputPortWidth=27  IndexOptions=Index vector (dialog)  Indices=[10]  OutputSizes=1
  balancingSelector11 : Selector  InputPortWidth=27  IndexOptions=Index vector (dialog)  Indices=[11]  OutputSizes=1
  balancingSelector12 : Selector  InputPortWidth=27  IndexOptions=Index vector (dialog)  Indices=[12]  OutputSizes=1
  balancingSelector13 : Selector  InputPortWidth=27  IndexOptions=Index vector (dialog)  Indices=[13]  OutputSizes=1
  balancingSelector14 : Selector  InputPortWidth=27  IndexOptions=Index vector (dialog)  Indices=[14]  OutputSizes=1
  balancingSelector15 : Selector  InputPortWidth=27  IndexOptions=Index vector (dialog)  Indices=[15]  OutputSizes=1
  balancingSelector16 : Selector  InputPortWidth=27  IndexOptions=Index vector (dialog)  Indices=[16]  OutputSizes=1
  balancingSelector17 : Selector  InputPortWidth=27  IndexOptions=Index vector (dialog)  Indices=[17]  OutputSizes=1
  balancingSelector18 : Selector  InputPortWidth=27  IndexOptions=Index vector (dialog)  Indices=[18]  OutputSizes=1
  balancingSelector19 : Selector  InputPortWidth=27  IndexOptions=Index vector (dialog)  Indices=[19]  OutputSizes=1
  balancingSelector2 : Selector  InputPortWidth=27  IndexOptions=Index vector (dialog)  Indices=[2]  OutputSizes=1
  balancingSelector20 : Selector  InputPortWidth=27  IndexOptions=Index vector (dialog)  Indices=[20]  OutputSizes=1
  balancingSelector21 : Selector  InputPortWidth=27  IndexOptions=Index vector (dialog)  Indices=[21]  OutputSizes=1
  balancingSelector22 : Selector  InputPortWidth=27  IndexOptions=Index vector (dialog)  Indices=[22]  OutputSizes=1
  balancingSelector23 : Selector  InputPortWidth=27  IndexOptions=Index vector (dialog)  Indices=[23]  OutputSizes=1
  balancingSelector24 : Selector  InputPortWidth=27  IndexOptions=Index vector (dialog)  Indices=[24]  OutputSizes=1
  balancingSelector25 : Selector  InputPortWidth=27  IndexOptions=Index vector (dialog)  Indices=[25]  OutputSizes=1
  balancingSelector26 : Selector  InputPortWidth=27  IndexOptions=Index vector (dialog)  Indices=[26]  OutputSizes=1
  balancingSelector27 : Selector  InputPortWidth=27  IndexOptions=Index vector (dialog)  Indices=[27]  OutputSizes=1
  balancingSelector3 : Selector  InputPortWidth=27  IndexOptions=Index vector (dialog)  Indices=[3]  OutputSizes=1
  balancingSelector4 : Selector  InputPortWidth=27  IndexOptions=Index vector (dialog)  Indices=[4]  OutputSizes=1
  balancingSelector5 : Selector  InputPortWidth=27  IndexOptions=Index vector (dialog)  Indices=[5]  OutputSizes=1
  balancingSelector6 : Selector  InputPortWidth=27  IndexOptions=Index vector (dialog)  Indices=[6]  OutputSizes=1
  balancingSelector7 : Selector  InputPortWidth=27  IndexOptions=Index vector (dialog)  Indices=[7]  OutputSizes=1
  balancingSelector8 : Selector  InputPortWidth=27  IndexOptions=Index vector (dialog)  Indices=[8]  OutputSizes=1
  balancingSelector9 : Selector  InputPortWidth=27  IndexOptions=Index vector (dialog)  Indices=[9]  OutputSizes=1
  iCellMux : Mux  Inputs=27
  numCyclesCellMux : Mux  Inputs=27
  socCellMux : Mux  Inputs=27
  socParallelAssemblyMux : Mux  Inputs=27
  temperatureCellMux : Mux  Inputs=27
  vCellMux : Mux  Inputs=27
  vParallelAssemblyMux : Mux  Inputs=27
  + : PMIOPort  Side=Left
  - : PMIOPort  Port=2  Side=Right
  iCell : Outport
  numCyclesCell : Outport  Port=2
  socCell : Outport  Port=3
  socParallelAssembly : Outport  Port=4
  temperatureCell : Outport  Port=5
  vCell : Outport  Port=6
  vParallelAssembly : Outport  Port=7
  wires:
  balancingSelector27/1 -> [balancing27]
  [balancing27] -> Converter27/1
  balancingSelector26/1 -> [balancing26]
  [balancing26] -> Converter26/1
  balancingSelector25/1 -> [balancing25]
  [balancing25] -> Converter25/1
  balancingSelector24/1 -> [balancing24]
  [balancing24] -> Converter24/1
  balancingSelector23/1 -> [balancing23]
  [balancing23] -> Converter23/1
  balancingSelector22/1 -> [balancing22]
  [balancing22] -> Converter22/1
  balancingSelector21/1 -> [balancing21]
  [balancing21] -> Converter21/1
  balancingSelector20/1 -> [balancing20]
  [balancing20] -> Converter20/1
  balancingSelector19/1 -> [balancing19]
  [balancing19] -> Converter19/1
  balancingSelector18/1 -> [balancing18]
  [balancing18] -> Converter18/1
  balancingSelector17/1 -> [balancing17]
  [balancing17] -> Converter17/1
  balancingSelector16/1 -> [balancing16]
  [balancing16] -> Converter16/1
  balancingSelector15/1 -> [balancing15]
  [balancing15] -> Converter15/1
  balancingSelector14/1 -> [balancing14]
  [balancing14] -> Converter14/1
  balancingSelector13/1 -> [balancing13]
  [balancing13] -> Converter13/1
  balancingSelector12/1 -> [balancing12]
  [balancing12] -> Converter12/1
  balancingSelector11/1 -> [balancing11]
  [balancing11] -> Converter11/1
  balancingSelector10/1 -> [balancing10]
  [balancing10] -> Converter10/1
  balancingSelector9/1 -> [balancing9]
  [balancing9] -> Converter9/1
  balancingSelector8/1 -> [balancing8]
  [balancing8] -> Converter8/1
  balancingSelector7/1 -> [balancing7]
  [balancing7] -> Converter7/1
  balancingSelector6/1 -> [balancing6]
  [balancing6] -> Converter6/1
  balancingSelector5/1 -> [balancing5]
  [balancing5] -> Converter5/1
  balancingSelector4/1 -> [balancing4]
  [balancing4] -> Converter4/1
  balancingSelector3/1 -> [balancing3]
  [balancing3] -> Converter3/1
  balancingSelector2/1 -> [balancing2]
  [balancing2] -> Converter2/1
  balancingSelector1/1 -> [balancing1]
  balancing/1 -> balancingSelector27/1, balancingSelector26/1, balancingSelector25/1, balancingSelector24/1, balancingSelector23/1, balancingSelector22/1, balancingSelector21/1, balancingSelector20/1, balancingSelector19/1, balancingSelector18/1, balancingSelector17/1, balancingSelector16/1, balancingSelector15/1, balancingSelector14/1, balancingSelector13/1, balancingSelector12/1, balancingSelector11/1, balancingSelector10/1, balancingSelector9/1, balancingSelector8/1, balancingSelector7/1, balancingSelector6/1, balancingSelector5/1, balancingSelector4/1, balancingSelector3/1, balancingSelector2/1, balancingSelector1/1
  [balancing1] -> Converter1/1
  [vParallelAssembly27] -> vParallelAssemblyMux/27
  Module27_outputs/7 -> [vParallelAssembly27]
  [vCell27] -> vCellMux/27
  Module27_outputs/6 -> [vCell27]
  [temperatureCell27] -> temperatureCellMux/27
  Module27_outputs/5 -> [temperatureCell27]
  [socParallelAssembly27] -> socParallelAssemblyMux/27
  Module27_outputs/4 -> [socParallelAssembly27]
  [socCell27] -> socCellMux/27
  Module27_outputs/3 -> [socCell27]
  [numCyclesCell27] -> numCyclesCellMux/27
  Module27_outputs/2 -> [numCyclesCell27]
  [iCell27] -> iCellMux/27
  Module27_outputs/1 -> [iCell27]
  [vParallelAssembly26] -> vParallelAssemblyMux/26
  Module26_outputs/7 -> [vParallelAssembly26]
  [vCell26] -> vCellMux/26
  Module26_outputs/6 -> [vCell26]
  [temperatureCell26] -> temperatureCellMux/26
  Module26_outputs/5 -> [temperatureCell26]
  [socParallelAssembly26] -> socParallelAssemblyMux/26
  Module26_outputs/4 -> [socParallelAssembly26]
  [socCell26] -> socCellMux/26
  Module26_outputs/3 -> [socCell26]
  [numCyclesCell26] -> numCyclesCellMux/26
  Module26_outputs/2 -> [numCyclesCell26]
  [iCell26] -> iCellMux/26
  Module26_outputs/1 -> [iCell26]
  [vParallelAssembly25] -> vParallelAssemblyMux/25
  Module25_outputs/7 -> [vParallelAssembly25]
  [vCell25] -> vCellMux/25
  Module25_outputs/6 -> [vCell25]
  [temperatureCell25] -> temperatureCellMux/25
  Module25_outputs/5 -> [temperatureCell25]
  [socParallelAssembly25] -> socParallelAssemblyMux/25
  Module25_outputs/4 -> [socParallelAssembly25]
  [socCell25] -> socCellMux/25
  Module25_outputs/3 -> [socCell25]
  [numCyclesCell25] -> numCyclesCellMux/25
  Module25_outputs/2 -> [numCyclesCell25]
  [iCell25] -> iCellMux/25
  Module25_outputs/1 -> [iCell25]
  [vParallelAssembly24] -> vParallelAssemblyMux/24
  Module24_outputs/7 -> [vParallelAssembly24]
  [vCell24] -> vCellMux/24
  Module24_outputs/6 -> [vCell24]
  [temperatureCell24] -> temperatureCellMux/24
  Module24_outputs/5 -> [temperatureCell24]
  [socParallelAssembly24] -> socParallelAssemblyMux/24
  Module24_outputs/4 -> [socParallelAssembly24]
  [socCell24] -> socCellMux/24
  Module24_outputs/3 -> [socCell24]
  [numCyclesCell24] -> numCyclesCellMux/24
  Module24_outputs/2 -> [numCyclesCell24]
  [iCell24] -> iCellMux/24
  Module24_outputs/1 -> [iCell24]
  [vParallelAssembly23] -> vParallelAssemblyMux/23
  Module23_outputs/7 -> [vParallelAssembly23]
  [vCell23] -> vCellMux/23
  Module23_outputs/6 -> [vCell23]
  [temperatureCell23] -> temperatureCellMux/23
  Module23_outputs/5 -> [temperatureCell23]
  [socParallelAssembly23] -> socParallelAssemblyMux/23
  Module23_outputs/4 -> [socParallelAssembly23]
  [socCell23] -> socCellMux/23
  Module23_outputs/3 -> [socCell23]
  [numCyclesCell23] -> numCyclesCellMux/23
  Module23_outputs/2 -> [numCyclesCell23]
  [iCell23] -> iCellMux/23
  Module23_outputs/1 -> [iCell23]
  [vParallelAssembly22] -> vParallelAssemblyMux/22
  Module22_outputs/7 -> [vParallelAssembly22]
  [vCell22] -> vCellMux/22
  Module22_outputs/6 -> [vCell22]
  [temperatureCell22] -> temperatureCellMux/22
  Module22_outputs/5 -> [temperatureCell22]
  [socParallelAssembly22] -> socParallelAssemblyMux/22
  Module22_outputs/4 -> [socParallelAssembly22]
  [socCell22] -> socCellMux/22
  Module22_outputs/3 -> [socCell22]
  [numCyclesCell22] -> numCyclesCellMux/22
  Module22_outputs/2 -> [numCyclesCell22]
  [iCell22] -> iCellMux/22
  Module22_outputs/1 -> [iCell22]
  [vParallelAssembly21] -> vParallelAssemblyMux/21
  Module21_outputs/7 -> [vParallelAssembly21]
  [vCell21] -> vCellMux/21
  Module21_outputs/6 -> [vCell21]
  [temperatureCell21] -> temperatureCellMux/21
  Module21_outputs/5 -> [temperatureCell21]
  [socParallelAssembly21] -> socParallelAssemblyMux/21
  Module21_outputs/4 -> [socParallelAssembly21]
  [socCell21] -> socCellMux/21
  Module21_outputs/3 -> [socCell21]
  [numCyclesCell21] -> numCyclesCellMux/21
  Module21_outputs/2 -> [numCyclesCell21]
  [iCell21] -> iCellMux/21
  Module21_outputs/1 -> [iCell21]
  [vParallelAssembly20] -> vParallelAssemblyMux/20
  Module20_outputs/7 -> [vParallelAssembly20]
  [vCell20] -> vCellMux/20
  Module20_outputs/6 -> [vCell20]
  [temperatureCell20] -> temperatureCellMux/20
  Module20_outputs/5 -> [temperatureCell20]
  [socParallelAssembly20] -> socParallelAssemblyMux/20
  Module20_outputs/4 -> [socParallelAssembly20]
  [socCell20] -> socCellMux/20
  Module20_outputs/3 -> [socCell20]
  [numCyclesCell20] -> numCyclesCellMux/20
  Module20_outputs/2 -> [numCyclesCell20]
  [iCell20] -> iCellMux/20
  Module20_outputs/1 -> [iCell20]
  [vParallelAssembly19] -> vParallelAssemblyMux/19
  Module19_outputs/7 -> [vParallelAssembly19]
  [vCell19] -> vCellMux/19
  Module19_outputs/6 -> [vCell19]
  [temperatureCell19] -> temperatureCellMux/19
  Module19_outputs/5 -> [temperatureCell19]
  [socParallelAssembly19] -> socParallelAssemblyMux/19
  Module19_outputs/4 -> [socParallelAssembly19]
  [socCell19] -> socCellMux/19
  Module19_outputs/3 -> [socCell19]
  [numCyclesCell19] -> numCyclesCellMux/19
  Module19_outputs/2 -> [numCyclesCell19]
  [iCell19] -> iCellMux/19
  Module19_outputs/1 -> [iCell19]
  [vParallelAssembly18] -> vParallelAssemblyMux/18
  Module18_outputs/7 -> [vParallelAssembly18]
  [vCell18] -> vCellMux/18
  Module18_outputs/6 -> [vCell18]
  [temperatureCell18] -> temperatureCellMux/18
  Module18_outputs/5 -> [temperatureCell18]
  [socParallelAssembly18] -> socParallelAssemblyMux/18
  Module18_outputs/4 -> [socParallelAssembly18]
  [socCell18] -> socCellMux/18
  Module18_outputs/3 -> [socCell18]
  [numCyclesCell18] -> numCyclesCellMux/18
  Module18_outputs/2 -> [numCyclesCell18]
  [iCell18] -> iCellMux/18
  Module18_outputs/1 -> [iCell18]
  [vParallelAssembly17] -> vParallelAssemblyMux/17
  Module17_outputs/7 -> [vParallelAssembly17]
  [vCell17] -> vCellMux/17
  Module17_outputs/6 -> [vCell17]
  [temperatureCell17] -> temperatureCellMux/17
  Module17_outputs/5 -> [temperatureCell17]
  [socParallelAssembly17] -> socParallelAssemblyMux/17
  Module17_outputs/4 -> [socParallelAssembly17]
  [socCell17] -> socCellMux/17
  Module17_outputs/3 -> [socCell17]
  [numCyclesCell17] -> numCyclesCellMux/17
  Module17_outputs/2 -> [numCyclesCell17]
  [iCell17] -> iCellMux/17
  Module17_outputs/1 -> [iCell17]
  [vParallelAssembly16] -> vParallelAssemblyMux/16
  Module16_outputs/7 -> [vParallelAssembly16]
  [vCell16] -> vCellMux/16
  Module16_outputs/6 -> [vCell16]
  [temperatureCell16] -> temperatureCellMux/16
  Module16_outputs/5 -> [temperatureCell16]
  [socParallelAssembly16] -> socParallelAssemblyMux/16
  Module16_outputs/4 -> [socParallelAssembly16]
  [socCell16] -> socCellMux/16
  Module16_outputs/3 -> [socCell16]
  [numCyclesCell16] -> numCyclesCellMux/16
  Module16_outputs/2 -> [numCyclesCell16]
  [iCell16] -> iCellMux/16
  Module16_outputs/1 -> [iCell16]
  [vParallelAssembly15] -> vParallelAssemblyMux/15
  Module15_outputs/7 -> [vParallelAssembly15]
  [vCell15] -> vCellMux/15
  Module15_outputs/6 -> [vCell15]
  [temperatureCell15] -> temperatureCellMux/15
  Module15_outputs/5 -> [temperatureCell15]
  [socParallelAssembly15] -> socParallelAssemblyMux/15
  Module15_outputs/4 -> [socParallelAssembly15]
  [socCell15] -> socCellMux/15
  Module15_outputs/3 -> [socCell15]
  [numCyclesCell15] -> numCyclesCellMux/15
  Module15_outputs/2 -> [numCyclesCell15]
  [iCell15] -> iCellMux/15
  Module15_outputs/1 -> [iCell15]
  [vParallelAssembly14] -> vParallelAssemblyMux/14
  Module14_outputs/7 -> [vParallelAssembly14]
  [vCell14] -> vCellMux/14
  Module14_outputs/6 -> [vCell14]
  [temperatureCell14] -> temperatureCellMux/14
  Module14_outputs/5 -> [temperatureCell14]
  [socParallelAssembly14] -> socParallelAssemblyMux/14
  Module14_outputs/4 -> [socParallelAssembly14]
  [socCell14] -> socCellMux/14
  Module14_outputs/3 -> [socCell14]
  [numCyclesCell14] -> numCyclesCellMux/14
  Module14_outputs/2 -> [numCyclesCell14]
  [iCell14] -> iCellMux/14
  Module14_outputs/1 -> [iCell14]
  [vParallelAssembly13] -> vParallelAssemblyMux/13
  Module13_outputs/7 -> [vParallelAssembly13]
  [vCell13] -> vCellMux/13
  Module13_outputs/6 -> [vCell13]
  [temperatureCell13] -> temperatureCellMux/13
  Module13_outputs/5 -> [temperatureCell13]
  [socParallelAssembly13] -> socParallelAssemblyMux/13
  Module13_outputs/4 -> [socParallelAssembly13]
  [socCell13] -> socCellMux/13
  Module13_outputs/3 -> [socCell13]
  [numCyclesCell13] -> numCyclesCellMux/13
  Module13_outputs/2 -> [numCyclesCell13]
  [iCell13] -> iCellMux/13
  Module13_outputs/1 -> [iCell13]
  [vParallelAssembly12] -> vParallelAssemblyMux/12
  Module12_outputs/7 -> [vParallelAssembly12]
  [vCell12] -> vCellMux/12
  Module12_outputs/6 -> [vCell12]
  [temperatureCell12] -> temperatureCellMux/12
  Module12_outputs/5 -> [temperatureCell12]
  [socParallelAssembly12] -> socParallelAssemblyMux/12
  Module12_outputs/4 -> [socParallelAssembly12]
  [socCell12] -> socCellMux/12
  Module12_outputs/3 -> [socCell12]
  [numCyclesCell12] -> numCyclesCellMux/12
  Module12_outputs/2 -> [numCyclesCell12]
  [iCell12] -> iCellMux/12
  Module12_outputs/1 -> [iCell12]
  [vParallelAssembly11] -> vParallelAssemblyMux/11
  Module11_outputs/7 -> [vParallelAssembly11]
  [vCell11] -> vCellMux/11
  Module11_outputs/6 -> [vCell11]
  [temperatureCell11] -> temperatureCellMux/11
  Module11_outputs/5 -> [temperatureCell11]
  [socParallelAssembly11] -> socParallelAssemblyMux/11
  Module11_outputs/4 -> [socParallelAssembly11]
  [socCell11] -> socCellMux/11
  Module11_outputs/3 -> [socCell11]
  [numCyclesCell11] -> numCyclesCellMux/11
  Module11_outputs/2 -> [numCyclesCell11]
  [iCell11] -> iCellMux/11
  Module11_outputs/1 -> [iCell11]
  [vParallelAssembly10] -> vParallelAssemblyMux/10
  Module10_outputs/7 -> [vParallelAssembly10]
  [vCell10] -> vCellMux/10
  Module10_outputs/6 -> [vCell10]
  [temperatureCell10] -> temperatureCellMux/10
  Module10_outputs/5 -> [temperatureCell10]
  [socParallelAssembly10] -> socParallelAssemblyMux/10
  Module10_outputs/4 -> [socParallelAssembly10]
  [socCell10] -> socCellMux/10
  Module10_outputs/3 -> [socCell10]
  [numCyclesCell10] -> numCyclesCellMux/10
  Module10_outputs/2 -> [numCyclesCell10]
  [iCell10] -> iCellMux/10
  Module10_outputs/1 -> [iCell10]
  [vParallelAssembly9] -> vParallelAssemblyMux/9
  Module09_outputs/7 -> [vParallelAssembly9]
  [vCell9] -> vCellMux/9
  Module09_outputs/6 -> [vCell9]
  [temperatureCell9] -> temperatureCellMux/9
  Module09_outputs/5 -> [temperatureCell9]
  [socParallelAssembly9] -> socParallelAssemblyMux/9
  Module09_outputs/4 -> [socParallelAssembly9]
  [socCell9] -> socCellMux/9
  Module09_outputs/3 -> [socCell9]
  [numCyclesCell9] -> numCyclesCellMux/9
  Module09_outputs/2 -> [numCyclesCell9]
  [iCell9] -> iCellMux/9
  Module09_outputs/1 -> [iCell9]
  [vParallelAssembly8] -> vParallelAssemblyMux/8
  Module08_outputs/7 -> [vParallelAssembly8]
  [vCell8] -> vCellMux/8
  Module08_outputs/6 -> [vCell8]
  [temperatureCell8] -> temperatureCellMux/8
  Module08_outputs/5 -> [temperatureCell8]
  [socParallelAssembly8] -> socParallelAssemblyMux/8
  Module08_outputs/4 -> [socParallelAssembly8]
  [socCell8] -> socCellMux/8
  Module08_outputs/3 -> [socCell8]
  [numCyclesCell8] -> numCyclesCellMux/8
  Module08_outputs/2 -> [numCyclesCell8]
  [iCell8] -> iCellMux/8
  Module08_outputs/1 -> [iCell8]
  [vParallelAssembly7] -> vParallelAssemblyMux/7
  Module07_outputs/7 -> [vParallelAssembly7]
  [vCell7] -> vCellMux/7
  Module07_outputs/6 -> [vCell7]
  [temperatureCell7] -> temperatureCellMux/7
  Module07_outputs/5 -> [temperatureCell7]
  [socParallelAssembly7] -> socParallelAssemblyMux/7
  Module07_outputs/4 -> [socParallelAssembly7]
  [socCell7] -> socCellMux/7
  Module07_outputs/3 -> [socCell7]
  [numCyclesCell7] -> numCyclesCellMux/7
  Module07_outputs/2 -> [numCyclesCell7]
  [iCell7] -> iCellMux/7
  Module07_outputs/1 -> [iCell7]
  [vParallelAssembly6] -> vParallelAssemblyMux/6
  Module06_outputs/7 -> [vParallelAssembly6]
  [vCell6] -> vCellMux/6
  Module06_outputs/6 -> [vCell6]
  [temperatureCell6] -> temperatureCellMux/6
  Module06_outputs/5 -> [temperatureCell6]
  [socParallelAssembly6] -> socParallelAssemblyMux/6
  Module06_outputs/4 -> [socParallelAssembly6]
  [socCell6] -> socCellMux/6
  Module06_outputs/3 -> [socCell6]
  [numCyclesCell6] -> numCyclesCellMux/6
  Module06_outputs/2 -> [numCyclesCell6]
  [iCell6] -> iCellMux/6
  Module06_outputs/1 -> [iCell6]
  [vParallelAssembly5] -> vParallelAssemblyMux/5
  Module05_outputs/7 -> [vParallelAssembly5]
  [vCell5] -> vCellMux/5
  Module05_outputs/6 -> [vCell5]
  [temperatureCell5] -> temperatureCellMux/5
  Module05_outputs/5 -> [temperatureCell5]
  [socParallelAssembly5] -> socParallelAssemblyMux/5
  Module05_outputs/4 -> [socParallelAssembly5]
  [socCell5] -> socCellMux/5
  Module05_outputs/3 -> [socCell5]
  [numCyclesCell5] -> numCyclesCellMux/5
  Module05_outputs/2 -> [numCyclesCell5]
  [iCell5] -> iCellMux/5
  Module05_outputs/1 -> [iCell5]
  [vParallelAssembly4] -> vParallelAssemblyMux/4
  Module04_outputs/7 -> [vParallelAssembly4]
  [vCell4] -> vCellMux/4
  Module04_outputs/6 -> [vCell4]
  [temperatureCell4] -> temperatureCellMux/4
  Module04_outputs/5 -> [temperatureCell4]
  [socParallelAssembly4] -> socParallelAssemblyMux/4
  Module04_outputs/4 -> [socParallelAssembly4]
  [socCell4] -> socCellMux/4
  Module04_outputs/3 -> [socCell4]
  [numCyclesCell4] -> numCyclesCellMux/4
  Module04_outputs/2 -> [numCyclesCell4]
  [iCell4] -> iCellMux/4
  Module04_outputs/1 -> [iCell4]
  [vParallelAssembly3] -> vParallelAssemblyMux/3
  Module03_outputs/7 -> [vParallelAssembly3]
  [vCell3] -> vCellMux/3
  Module03_outputs/6 -> [vCell3]
  [temperatureCell3] -> temperatureCellMux/3
  Module03_outputs/5 -> [temperatureCell3]
  [socParallelAssembly3] -> socParallelAssemblyMux/3
  Module03_outputs/4 -> [socParallelAssembly3]
  [socCell3] -> socCellMux/3
  Module03_outputs/3 -> [socCell3]
  [numCyclesCell3] -> numCyclesCellMux/3
  Module03_outputs/2 -> [numCyclesCell3]
  [iCell3] -> iCellMux/3
  Module03_outputs/1 -> [iCell3]
  [vParallelAssembly2] -> vParallelAssemblyMux/2
  Module02_outputs/7 -> [vParallelAssembly2]
  [vCell2] -> vCellMux/2
  Module02_outputs/6 -> [vCell2]
  [temperatureCell2] -> temperatureCellMux/2
  Module02_outputs/5 -> [temperatureCell2]
  [socParallelAssembly2] -> socParallelAssemblyMux/2
  Module02_outputs/4 -> [socParallelAssembly2]
  [socCell2] -> socCellMux/2
  Module02_outputs/3 -> [socCell2]
  [numCyclesCell2] -> numCyclesCellMux/2
  Module02_outputs/2 -> [numCyclesCell2]
  [iCell2] -> iCellMux/2
  Module02_outputs/1 -> [iCell2]
  [vParallelAssembly1] -> vParallelAssemblyMux/1
  vParallelAssemblyMux/1 -> vParallelAssembly/1
  Module01_outputs/7 -> [vParallelAssembly1]
  [vCell1] -> vCellMux/1
  vCellMux/1 -> vCell/1
  Module01_outputs/6 -> [vCell1]
  [temperatureCell1] -> temperatureCellMux/1
  temperatureCellMux/1 -> temperatureCell/1
  Module01_outputs/5 -> [temperatureCell1]
  [socParallelAssembly1] -> socParallelAssemblyMux/1
  socParallelAssemblyMux/1 -> socParallelAssembly/1
  Module01_outputs/4 -> [socParallelAssembly1]
  [socCell1] -> socCellMux/1
  socCellMux/1 -> socCell/1
  Module01_outputs/3 -> [socCell1]
  [numCyclesCell1] -> numCyclesCellMux/1
  numCyclesCellMux/1 -> numCyclesCell/1
  Module01_outputs/2 -> [numCyclesCell1]
  [iCell1] -> iCellMux/1
  iCellMux/1 -> iCell/1
  Module01_outputs/1 -> [iCell1]
  connections:
  Converter27/RConn1 -- Module27/LConn1
  Converter26/RConn1 -- Module26/LConn1
  Converter25/RConn1 -- Module25/LConn1
  Converter24/RConn1 -- Module24/LConn1
  Converter23/RConn1 -- Module23/LConn1
  Converter22/RConn1 -- Module22/LConn1
  Converter21/RConn1 -- Module21/LConn1
  Converter20/RConn1 -- Module20/LConn1
  Converter19/RConn1 -- Module19/LConn1
  Converter18/RConn1 -- Module18/LConn1
  Converter17/RConn1 -- Module17/LConn1
  Converter16/RConn1 -- Module16/LConn1
  Converter15/RConn1 -- Module15/LConn1
  Converter14/RConn1 -- Module14/LConn1
  Converter13/RConn1 -- Module13/LConn1
  Converter12/RConn1 -- Module12/LConn1
  Converter11/RConn1 -- Module11/LConn1
  Converter10/RConn1 -- Module10/LConn1
  Converter9/RConn1 -- Module09/LConn1
  Converter8/RConn1 -- Module08/LConn1
  Converter7/RConn1 -- Module07/LConn1
  Converter6/RConn1 -- Module06/LConn1
  Converter5/RConn1 -- Module05/LConn1
  Converter4/RConn1 -- Module04/LConn1
  Converter3/RConn1 -- Module03/LConn1
  Converter2/RConn1 -- Module02/LConn1
  Converter1/RConn1 -- Module01/LConn1
  Module27/RConn1 -- -/RConn1
  Module01/LConn2 -- +/RConn1
  Module27/LConn2 -- Module26/RConn1
  Module26/LConn2 -- Module25/RConn1
  Module25/LConn2 -- Module24/RConn1
  Module24/LConn2 -- Module23/RConn1
  Module23/LConn2 -- Module22/RConn1
  Module22/LConn2 -- Module21/RConn1
  Module21/LConn2 -- Module20/RConn1
  Module20/LConn2 -- Module19/RConn1
  Module19/LConn2 -- Module18/RConn1
  Module18/LConn2 -- Module17/RConn1
  Module17/LConn2 -- Module16/RConn1
  Module16/LConn2 -- Module15/RConn1
  Module15/LConn2 -- Module14/RConn1
  Module14/LConn2 -- Module13/RConn1
  Module13/LConn2 -- Module12/RConn1
  Module12/LConn2 -- Module11/RConn1
  Module11/LConn2 -- Module10/RConn1
  Module10/LConn2 -- Module09/RConn1
  Module09/LConn2 -- Module08/RConn1
  Module08/LConn2 -- Module07/RConn1
  Module07/LConn2 -- Module06/RConn1
  Module06/LConn2 -- Module05/RConn1
  Module05/LConn2 -- Module04/RConn1
  Module04/LConn2 -- Module03/RConn1
  Module03/LConn2 -- Module02/RConn1
  Module02/LConn2 -- Module01/RConn1
